simulink model "model"  (R2018a)
settings: Solver=FixedStepDiscrete  StartTime=0.0  StopTime=10  FixedStep=Ts  RelTol=1e-3  EnableMultiTasking=on
undefined symbols (not defined in the file): AL, Cd, cr1, cr2, DiscIntNeverNeededParam, g, i_t, Ld, Lq, Mv, p, Pmax, psim, rho_a, Rs, Rw, sigbuilder_block, Tmax, Ts, Tsi, Tso, VDC_VECT, wmax
libraries: fl_lib x42, nesl_utility x16, pe_lib x5, simulink x3, pePmsmCurrentReferenceGen x3, peTransforms x2, simulink_extras x2, dspstat3 x2, pePmsmCurrentController x1, peDiscretePi x1, pePmsmFwController x1, pePmsmTorqueEstimator x1
(part 2 of 2)

== system model/Drive Controller/EM Controller/Outer Loop Control/MyFW/Prevent division by 0 ==
  IN : Inport
  Constant1 : Constant  Value=0.1  SampleTime=-1
  Switch : Switch  Criteria=u2 > Threshold  Threshold=0.1
  OUT : Outport
  wires:
  Switch/1 -> OUT/1
  IN/1 -> Switch/2, Switch/1
  Constant1/1 -> Switch/3

== system model/Drive Controller/EM Controller/Outer Loop Control/MyFW/Modulation index/Prevent division by 0 ==
  IN : Inport
  Constant1 : Constant  Value=0.1  SampleTime=-1
  Switch : Switch  Criteria=u2 > Threshold  Threshold=0.1
  OUT : Outport
  wires:
  Switch/1 -> OUT/1
  IN/1 -> Switch/2, Switch/1
  Constant1/1 -> Switch/3

== matlab function model/Drive Controller/EM Controller/Outer Loop Control/MATLAB Function1 ==
  data: Tref input; w input; idqRef output; wBase input; vdc input
function idqRef = myFieldWeakening(Tref, w, wBase, vdc)

%% Constants
Pmax = 2000e3;      % Maximum power                   [W]
Tmax = 5000;        % Maximum torque                  [N*m]
Ld   = 0.00024368; % Stator d-axis inductance        [H]
Lq   = 0.00029758; % Stator q-axis inductance        [H]
L0   = 0.00012184; % Stator zero-sequence inductance [H]
Rs   = 0.026;   % Stator resistance per phase     [Ohm]
psim = 0.1014;    % Permanent magnet flux linkage   [Wb]
p    = 10;          % Number of pole pairs

i_max = 200;

%% Data conversion
we = w*p;
we_base = wBase*p;
vs = vdc/sqrt(3);
vph_max = 650/sqrt(3);
k=0.997;

%% Controller
M = vs/(k*vph_max);
if w <= wBase || wBase < 0 %M <= 1
    disp('yeah?')
    disp([w, wBase])
    poly = [9*p^2*(Lq-Ld)^2, 0, 0, 6*Tref*p*psim, -4*Tref^2];
    iq = roots(poly);

    % Solve for id
    id = psim/(2*(Lq-Ld)) - sqrt(psim^2/(4*(Lq-Ld)^2)+iq.^2);
    
    Id_ref = real(id(4));
    Iq_ref = real(iq(4));
else
    disp('nup')
    disp(M)
    % Find roots of d-q torque equation (polynomial in terms of iq)
    poly = [9*p^2*(Lq-Ld)^2*Lq^2*we^2, 0, 9*p^2*psim^2*Lq^2*we^2 - 9*p^2*(Ld-Lq)^2*vph_max^2, -12*Tref*p*psim*Ld*Lq*we^2, 4*Tref^2*Ld^2*we^2];
    iq_fw = roots(poly);

    % Solve for id
    id_fw = -psim/Ld + (1/Ld)*sqrt((vph_max^2)/(we^2)-(Lq*iq_fw).^2);
    
    disp('iq_fw=')
    disp(iq_fw);
    disp('id_fw=')
    disp(id_fw);
    disp('----')
    
    Id_ref = real(id_fw(1));
    Iq_ref = real(iq_fw(1));
end

idqRef = [Id_ref; Iq_ref];

%% Controller https://au.mathworks.com/help/mcb/ref/mtpacontrolreference.html
% k = 1;
% vmax = 650/sqrt(3);
% 
% im_ref = 2*Tref / (3*p*psim);
% im = max(im_ref, i_max);
% 
% if w <= k*wBase || w == 0
%     disp('.1.')
%     disp(psim/(4*(Lq-Ld)));
%     disp(psim^2/(16*(Lq-Ld)^2) + im^2/2);
%     disp(psim/(4*(Lq-Ld)) - sqrt(psim^2/(16*(Lq-Ld)^2) + im^2/2));
%     
%     id_mtpa = psim/(4*(Lq-Ld)) - sqrt(psim^2/(16*(Lq-Ld)^2) + im^2/2);
%     iq_mtpa = sqrt(im^2-id_mtpa^2);
% 
%     Id_ref = id_mtpa;
%     Iq_ref = iq_mtpa;
% else
%     disp('w:')
%     disp(w);
%     disp(k*wBase);
%     id_fw = (-psim*Ld+sqrt((psim*Ld)^2-(Ld^2-Lq^2)*(psim^2+Lq^2*i_max^2-vmax^2/we^2)))/(Ld^2-Lq^2);
%     iq_fw = sqrt(i_max^2-id_fw^2);
%     
%     Id_ref = max(id_fw, -i_max);
%     
%     if iq_fw < im
%         Iq_ref = iq_fw;
%     else
%         Iq_ref = im;
%     end
% end
% 
% idqRef = [Id_ref; Iq_ref];

== matlab function model/Drive Controller/EM Controller/Outer Loop Control/MATLAB Function ==
  data: Vdc input; w_base output; Rs input; Pmax input; Ldq input; idq input; psim input; rpm_base output; p input
function [w_base, rpm_base] = calcBaseSpeed(Vdc,Rs,Pmax,Ldq,idq,psim,p)
%calcBaseSpeed Calculates motor base speed
i_max = sqrt(3)*Pmax/Vdc;
v_max = max(Vdc/sqrt(3) - Rs*i_max, 0);

Ld = Ldq(1);
Lq = Ldq(2);
id = idq(1);
iq = idq(2);

w_base = (1/p)* v_max/sqrt((Lq*iq)^2+(Ld*id+psim)^2);
rpm_base = w_base * 30/pi;

end

== matlab function model/Drive Controller/EM Controller/Outer Loop Control/MATLAB Function2 ==
  data: Tref input; w input; idqRef output; wBase input; Vdc input; idqIn input
function idqRef = fwController(Tref, w, wBase, Vdc, idqIn)

%% Constants
Pmax = 2000e3;      % Maximum power                   [W]
Tmax = 5000;        % Maximum torque                  [N*m]
Ld   = 0.00024368; % Stator d-axis inductance        [H]
Lq   = 0.00029758; % Stator q-axis inductance        [H]
L0   = 0.00012184; % Stator zero-sequence inductance [H]
Rs   = 0.026;   % Stator resistance per phase     [Ohm]
psim = 0.1014;    % Permanent magnet flux linkage   [Wb]
p    = 10;          % Number of pole pairs

%% Data conversion
we = w*p;
we_base = wBase*p;

i_max = sqrt(3)*Pmax/Vdc;

eps = 1e-6; % Very small float

%% Controller https://au.mathworks.com/help/mcb/ref/mtpacontrolreference.html
k = 1;
vmax = 650/sqrt(3);

im_ref = 2*Tref / (3*p*psim);
im = max(im_ref, i_max);

if w <= k*wBase || w < eps
    disp('MTPA')
    disp(psim/(4*(Lq-Ld)));
    disp(psim^2/(16*(Lq-Ld)^2) + im^2/2);
    disp(psim/(4*(Lq-Ld)) - sqrt(psim^2/(16*(Lq-Ld)^2) + im^2/2));
    
    id_mtpa = psim/(4*(Lq-Ld)) - sqrt(psim^2/(16*(Lq-Ld)^2) + im^2/2);
    iq_mtpa = sqrt(im^2-id_mtpa^2);

    Id_ref = id_mtpa;
    Iq_ref = iq_mtpa;
else
    disp('FW, w:')
    disp(w);
    disp(k*wBase);
    id_fw = (-psim*Ld+sqrt((psim*Ld)^2-(Ld^2-Lq^2)*(psim^2+Lq^2*i_max^2-vmax^2/we^2)))/(Ld^2-Lq^2);
    disp(id_fw);
    iq_fw = sqrt(i_max^2-id_fw^2);
    
    Id_ref = max(id_fw, -i_max);
    
    if iq_fw < im
        Iq_ref = iq_fw;
    else
        Iq_ref = im;
    end
end

idqRef = [Id_ref; Iq_ref];
